simulink model "rotary_mass_spring_damper"  (R2019b)
settings: Solver=VariableStepAuto  StartTime=0.0  StopTime=10.0  RelTol=1e-3
model workspace (MAT data in the model file):
  B = 3
  J = 8.6
  dt = 0.01
  k = 10
undefined symbols (not defined in the file): NULL, serial
libraries: instrumentlib x3
settings Model: OrderedModelArguments=off  Creator=ctsai  LastModifiedBy=ctsai

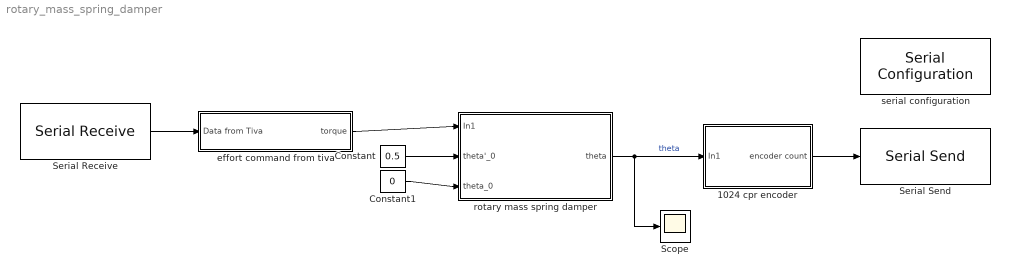
== system rotary_mass_spring_damper ==
  1024 cpr encoder : Subsystem
  Constant : Constant  Value=0.5
  Constant1 : Constant  Value=0
  Scope : Scope
  Serial Receive : instrumentlib/Serial Receive  ComPortMenu=COM4  ComPort=COM4  ObjConstructor=serial('COM4');  Terminator=NULL ('\0')  DataSize=[1 1]  DataType=int16  EnableBlockingMode=on  ActionDataUnavailable=Output last received value  CustomValue=0  SampleTime=dt
  Serial Send : instrumentlib/Serial Send  ComPortMenu=COM4  ComPort=COM4  ObjConstructor=serial('COM4');  Terminator=<none>  EnableBlockingMode=on
  effort command from tiva : Subsystem
  rotary mass spring damper : Subsystem
  serial configuration : instrumentlib/Serial Configuration  Priority=-200000  ComPortMenu=COM4  ComPort=COM4  ObjConstructor=serial('COM4');  BaudRate=115200  DataBits=8  Parity=none  StopBits=1  FlowControl=none  Timeout=10  ByteOrder=LittleEndian
  wires:
  effort command from tiva/1("torque ") -> rotary mass spring damper/1(In1)
  Constant/1 -> rotary mass spring damper/2(theta'_0)
  Constant1/1 -> rotary mass spring damper/3(theta_0)
  rotary mass spring damper/1(theta) -> Scope/1, 1024 cpr encoder/1(In1)  "theta"
  1024 cpr encoder/1(encoder count) -> Serial Send/1
  Serial Receive/1 -> effort command from tiva/1("Data from Tiva ")

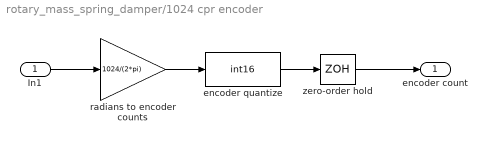
== system rotary_mass_spring_damper/1024 cpr encoder ==
  In1 : Inport
  encoder quantize : DataTypeConversion  OutDataTypeStr=int16
  radians to encoder counts : Gain  Gain=1024/(2*pi)
  zero-order hold : ZeroOrderHold  SampleTime=-1
  encoder count : Outport
  wires:
  radians to encoder counts/1 -> encoder quantize/1
  encoder quantize/1 -> zero-order hold/1
  zero-order hold/1 -> encoder count/1
  In1/1 -> radians to encoder counts/1

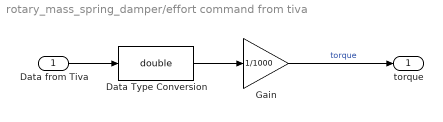
== system rotary_mass_spring_damper/effort command from tiva ==
  "Data from Tiva " : Inport
  Data Type Conversion : DataTypeConversion  OutDataTypeStr=double
  Gain : Gain  Gain=1/1000
  "torque " : Outport
  wires:
  Gain/1 -> "torque "/1  "torque"
  Data Type Conversion/1 -> Gain/1
  "Data from Tiva "/1 -> Data Type Conversion/1

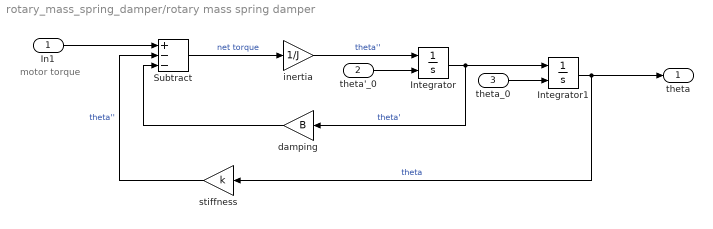
== system rotary_mass_spring_damper/rotary mass spring damper ==
  note: motor torque
  In1 : Inport
  theta'_0 : Inport  Port=2
  theta_0 : Inport  Port=3
  Integrator : Integrator  InitialConditionSource=external
  Integrator1 : Integrator  InitialConditionSource=external
  Subtract : Sum  Inputs=+--
  damping : Gain  Gain=B
  inertia : Gain  Gain=1/J
  stiffness : Gain  Gain=k
  theta : Outport
  wires:
  theta_0/1 -> Integrator1/2
  theta'_0/1 -> Integrator/2
  Subtract/1 -> inertia/1  "net torque"
  Integrator/1 -> damping/1, Integrator1/1  "theta'"
  damping/1 -> Subtract/3
  Integrator1/1 -> theta/1, stiffness/1  "theta"
  stiffness/1 -> Subtract/2  "theta''"
  inertia/1 -> Integrator/1  "theta''"
  In1/1 -> Subtract/1
